simulink model "system_FIR_bank_decoder"  (Simulink 8.3)
settings: Solver=ode45  StartTime=0.0  StopTime=10  RelTol=1e-3
undefined symbols (not defined in the file or in its folder): fdesignblkfcn, gcbh
libraries: commutil2 x2
(part 2 of 2)

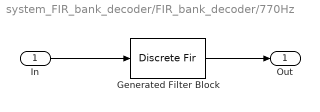
== system system_FIR_bank_decoder/FIR_bank_decoder/770Hz ==
  In : Inport
  Generated Filter Block : DiscreteFir  Tag=BlockMethodSubSystem  FilterStructure=Direct form symmetric  Coefficients=[0.021048100748084043 -0.02926286162127616 -0.014344339405233889 -0.0067382476342175519 -0.0033123904559366302 -0.0021945690276578204 -0.0021342071303361238 -0.0022934425052693599 -0.0021557510968869928 -0.001536841972853253 -0.0005235016935473541 0.00058759386859477594 0.0014491242644490197 0.0017708969698477183 0.0014585874915251354 0.00061878703844939242 -0.00044354826950585192 -0.00136089700455511 -0.0017988232627814934 -0.0016048306304633827 -0.00083332303586988873 0.0002421672794711616 0.0012517587307990547 0.001826200459492635 0.0017626470460959727 0.0010625791642325511 -2.6711098009971838e-05 -0.0011360179030814456 -0.0018571126120684983 -0.001935651064151669 -0.0013148457755932251 -0.00021185890996268823 0.0010052695934177559 0.0018872707487213719 0.0021248152733135744 0.0015951242710271173 0.00048699554077768256 -0.00084425051160600425 -0.0018964823074298872 -0.0023198333997277807 -0.0018939145551047107 -0.00080325835581027507 0.00064730516589957742 0.0018908439902302809 0.0024829039658738304 0.0022586425220235381 0.001118577978164267 -0.00038876585185248602 -0.0018239156066238533 -0.0026733845855196046 -0.0025850508415780015 -0.0015235746420565225 9.8462718731610923e-05 0.0017320698806078927 0.0028012826225293232 0.0029192523560542393 0.001972636913799473 0.0002734845029135913 -0.0015896954375363879 -0.0029233477215027909 -0.0032471603043519861 -0.0024101597386545605 -0.00068965280517628146 0.0013420758467165626 0.0029592478547132983 0.0035718941730886705 0.0029104506306473158 0.0011759708128102752 -0.0010476345159772472 -0.0029595495295805805 -0.0038642666267331735 -0.0033961128923412436 -0.0016942633995684863 0.00067242773425810838 0.0028625723334399292 0.0040920428977543402 0.003882971457832749 0.0022758252206261037 -0.00020302132854180453 -0.0026794330164426438 -0.0042706199501282589 -0.0043654735945765659 -0.0028983243153943477 -0.00033331843401783636 0.0024121533503752464 0.0043837819953542728 0.0048117339194579068 0.0035361082096169567 0.00094222332517836108 -0.0020601481562842537 -0.0043894290292150256 -0.005213252978909436 -0.0041781027657706582 -0.0016080612636526659 0.0015954691904100724 0.0043058302627674962 0.0055415888387755508 0.0048136835024899394 0.0023334413667720775 -0.0010362021330557435 -0.0041113741986643637 -0.0057862243907440408 -0.0054244151769606468 -0.0031030261300052128 0.00038481679566975817 0.0038081382852554664 0.0059389667376776919 0.0059894192755409513 0.0038935720589659611 0.00035523833276214235 -0.0033882281047023233 -0.005991540588728566 -0.0064993294746897032 -0.0046880882204626577 -0.0011646042858746047 0.0028465822396311108 0.0059164623818464962 0.0069265357518669985 0.0054720287743438879 0.0020301971526669846 -0.0022036194398257691 -0.0057212873206023158 -0.0072529382952613106 -0.0062136143169091882 -0.0029368435165044262 0.0014470907359265988 0.005384551681539747 0.0074587017277012273 0.0068995756468850332 0.0038548868599859731 -0.00061229573615546201 -0.0049387237433249449 -0.0075577428617720193 -0.007514679432755883 -0.0047852690650780341 -0.00030172072869157003 0.0043511265299573951 0.0075165351433368246 0.0080467150937750861 0.0057115794430851134 0.0013076313938961423 -0.0036156565354544738 -0.0073081930109354099 -0.0084400136036027733 -0.0065672305909212341 -0.0023245721628232432 0.0027968271489216224 0.0069794360967642098 0.00872015779915606 0.0073702080881285345 0.0033744958616032639 -0.0018647551369501331 -0.0064920262273558179 -0.0088511085597637752 -0.0080796097740328116 -0.0044191382710887022 0.00085345506904594228 0.0058715779690651079 0.0088409748695103384 0.0086860509306450791 0.0054356336329200059 0.00022143986170222401 -0.0051168645751970927 -0.0086748461106291707 -0.0091688916638644914 -0.0064015522032404909 -0.0013346529759097816 0.0042425490216516717 0.0083493712118810921 0.0095084847417085134 0.0072921448718452197 0.002465004547517967 -0.0032696589721588052 -0.00787137040913557 -0.0097013501466275687 -0.0080863506859156619 -0.0035909465012341248 ...(+5042 chars)]  InputProcessing=Columns as channels (frame based)
  Out : Outport
  wires:
  In/1 -> Generated Filter Block/1
  Generated Filter Block/1 -> Out/1

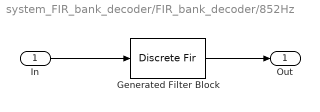
== system system_FIR_bank_decoder/FIR_bank_decoder/852Hz ==
  In : Inport
  Generated Filter Block : DiscreteFir  Tag=BlockMethodSubSystem  FilterStructure=Direct form symmetric  Coefficients=[0.023839593513569859 -0.026106670886814936 -0.014515913923892815 -0.0078635068286020057 -0.0045480316379694387 -0.0033125023745395172 -0.0030702773016210968 -0.0029641466005046573 -0.0024588534477011066 -0.0014330386067146878 -0.00011452378323294329 0.0010522474153322396 0.0016501906286755937 0.0014642374300596339 0.00060786967801007878 -0.00054209838800419775 -0.0014772482973398726 -0.0017921976058056773 -0.0013374155712994711 -0.00030506612887536638 0.00087472422424384356 0.0016866687577636987 0.0017817229796820561 0.0011008170041724777 -6.7951668830092398e-05 -0.0012338634266420179 -0.0018829581556778798 -0.0017310722292330893 -0.00081471251070362239 0.00047462403546293948 0.0015953679106102806 0.0020438242476589338 0.0016179295379949812 0.00046518805502698482 -0.00091654708573927243 -0.0019480212635727564 -0.0021464034237020165 -0.0014247206150643905 -3.7508109370541094e-05 0.0013906791174611499 0.0022706213384942465 0.0021899192012197204 0.0011001905319130917 -0.00042135809591145509 -0.0019045071189112523 -0.0025539731328647697 -0.002092463133230923 -0.00072009861981338775 0.0010000178906505223 0.0023770497455017541 0.0027529804807521294 0.0019202616543645158 0.00020435629835819638 -0.0016402729354980268 -0.0028262131054517343 -0.00281510525540949 -0.001583211314657491 0.00039262808518109873 0.0022694564801642417 0.0032224174937415602 0.0027848157683940233 0.0011074989164262419 -0.0011187022712652141 -0.0029195613294748721 -0.0034982347912125194 -0.0025584117004255574 -0.0004725215393152763 0.0018883392295170559 0.0034931229985446306 0.0036249270451743296 0.0021695195909299234 -0.00027888357370429843 -0.0026890375793498559 -0.0039958072741914418 -0.003597031588827398 -0.0016039092120171479 0.0011490864977044314 0.0034881849355724148 0.0043609149454591463 0.0033568320966274692 0.00083971336969076169 -0.0021067948801669501 -0.0042247171368122189 -0.0045502501148665933 -0.0028843693516404862 7.1967398731385661e-05 0.0030959780151318733 0.0048375524262719511 0.0045065369818951592 0.0022050002374939003 -0.0011215697125002667 -0.0040524937311592173 -0.0052801949618826649 -0.0042294902609412849 -0.0013093666776701719 0.0022536705603679683 0.0049270206978740223 0.0055144523843526656 0.0037058428394836007 0.0002355501063833989 -0.003415786161396827 -0.0056604358884984381 -0.0054892043449990078 -0.002920784864148521 0.00098471497505570656 0.0045496559355458384 0.0062074456351294436 0.0051917415254992003 0.0018893813508643899 -0.0023049838224737575 -0.0055797767405325197 -0.0064930396376156416 -0.0045954018879252453 -0.00065797037911517655 0.0036463250897162645 0.0064461224748369956 0.0064897427719319807 0.0037047375428177517 -0.00074460471538265606 -0.0049517196141328542 -0.0070744820626486475 -0.006158689233933555 -0.0025398425003342515 0.0022400377908260681 0.0061321131231064883 0.0074208299658351856 0.0054982560497843233 0.001156840977674564 -0.0037672796052483936 -0.0071289770683121961 -0.0074409759411050418 -0.0045249287379080828 0.00040422482224439075 0.0052351315586598411 0.0078578153585284211 0.0071062950474576865 0.0032608445674290544 -0.0020543345264128743 -0.0065522878586134672 -0.0082622360756481987 -0.0064084536760591389 -0.0017513523048681943 0.0037234866712307045 0.0076513455140711662 0.0083049672715876689 0.0053605338667787441 5.1003415149181457e-05 -0.0053414146508846995 -0.00847846955851159 -0.0079752044526672852 -0.0040080457338613424 0.0017406403995727327 0.0067924186865504525 0.0089517847692777534 0.0072490495502076386 0.0023900675486357285 -0.0035492195807516553 -0.0080034008198448317 -0.0090283068818453084 -0.0061482263646378699 -0.00057659715051141191 0.0052956996274064758 0.008921751675892188 0.0087164235545905654 0.0047329535394271607 -0.0013216208552966494 -0.0068503409744694278 -0.0094509499938668778 -0.0079763849798731006 -0.0030398229397014887 0.0032491107768218498 0.0081733712904150067 0.0095901393340554145 0.0068689647994716026 0.0011591458925277064 -0.005083069295184206 -0.0091558726262952802 ...(+5053 chars)]  InputProcessing=Columns as channels (frame based)
  Out : Outport
  wires:
  In/1 -> Generated Filter Block/1
  Generated Filter Block/1 -> Out/1

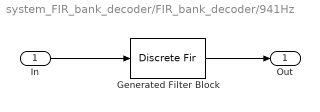
== system system_FIR_bank_decoder/FIR_bank_decoder/941Hz ==
  In : Inport
  Generated Filter Block : DiscreteFir  Tag=BlockMethodSubSystem  FilterStructure=Direct form symmetric  Coefficients=[0.025509633378811274 0.022027391281937769 -0.015629739982581058 0.01066284803954645 -0.0047831166861981292 0.0056878627848254123 -0.0019775559228465884 0.0012287487691349298 -0.0025670139817215295 -0.00089682443127405591 -0.0014324914095788913 0.00050888938642988039 0.0010653809095696922 0.0017962985083336011 0.0011208597776862796 0.00015952992258727708 -0.0010928572659544237 -0.0016584138927316103 -0.0014437839602567924 -0.00041506486813670373 0.00081415889396011182 0.0016601893507764819 0.0016336138422862543 0.00075543418376772622 -0.00054633853810124265 -0.0015869279553149694 -0.0018179488734876175 -0.0010935995063684118 0.0002287098190819126 0.0014648523119702398 0.0019647018619948432 0.001436416543403227 0.00013333133020686287 -0.0012817439544525135 -0.0020625248600068201 -0.0017768482585151014 -0.00053840721495798302 0.0010259408009693229 0.002099359380323892 0.0020903968392256421 0.00097089286371020275 -0.00071237104384959708 -0.0020702200555446438 -0.0023841595545743546 -0.0014492241416905142 0.00026574605147578482 0.0019094243426282453 0.0026117440970939744 0.0019437477009074892 0.00018307405317330571 -0.0017232791496264183 -0.0027566422826116386 -0.0023748863380560889 -0.0007350485104265801 0.0013836672211365495 0.0028332519276649142 0.0028108297305253749 0.0013174472467332816 -0.00092556264659052418 -0.0027826385279787064 -0.003201011718975369 -0.0019430086446150865 0.00037465411450848032 0.0025928002837349762 0.0035058400781362823 0.0025764007836806351 0.0002738990187042084 -0.0022695720481412168 -0.0036928074752020741 -0.0031870266537408873 -0.0009984174627757842 0.0018055402857457738 0.0037437476847058493 0.0037404939922762079 0.0017767189026404685 -0.0012058229600212691 -0.0036387020273276594 -0.0042045380891096995 -0.0025791591383506262 0.00048068760015451055 0.0033677770188416598 0.0045516701866640573 0.0033737188659410783 0.00035582322408828733 -0.0029178694320686886 -0.0047427881264862533 -0.0041115140023262496 -0.0012732346779163004 0.0023009278413217539 0.0047663412986232332 0.0047777260036137277 0.002253543599482365 -0.0015161883494841943 -0.0046015754267823717 -0.0053064217321209571 -0.0032372140061104667 0.00059142724660077957 0.0042051604868857196 0.0056766845822321475 0.0042018156960761926 0.00045171511976631551 -0.0036106993858542303 -0.005859781468159784 -0.0050775447330761317 -0.0015853396244687303 0.0028122744369163915 0.0058345648635002682 0.0058279044082092425 0.0027595622967925776 -0.0018328537806899094 -0.0055645182261874152 -0.0064236665849391394 -0.003925385001803978 0.00070013454311207706 0.0050431539301435254 0.0068180207947109743 0.0050311231388792035 0.00055595950578312282 -0.0042835843576532109 -0.0069750609934890288 -0.0060221129287031643 -0.001896624251093112 0.0033075635262751492 0.0068594085369391815 0.0068608579428576771 0.0032502975097536031 -0.0021319075260896121 -0.0064745520716545379 -0.0074940038004008887 -0.0045697271203565199 0.00078352658949030173 0.005820345492641303 0.0078682178156787227 0.0058072344641340295 0.00066912298961172348 -0.0049054770897861179 -0.0079698217689620626 -0.0068998037835217765 -0.002172008716647628 0.0037403534797150698 0.0077841828110188534 0.0077765126315403072 0.003698794600225258 -0.0023803062078963594 -0.0072885878984963208 -0.0084188750924269716 -0.005152502157324065 0.00086386672700348001 0.006489495104535406 0.0087789808308271645 0.0064792389847687223 0.00076217441800956534 -0.0054224346548773644 -0.0088146235301680403 -0.0076270280739622574 -0.0024244856601635164 0.0041053566776316349 0.0085308046712537829 0.0085368672595809367 0.0040564387482297324 -0.0025766252143383816 -0.0079289424423843423 -0.0091568569648412274 -0.0056065783056036631 0.00091675555196166388 0.0069992068855367785 0.0094768847001047499 0.0069880904510374077 0.00084457967604023609 -0.0058019139649227837 -0.0094385197591500703 -0.0081659172256053174 -0.0026052572843086688 0.0043467315054058295 0.0090666733847423724 0.0090679844972093356 0.0043234443682321471 ...(+5045 chars)]  InputProcessing=Columns as channels (frame based)
  Out : Outport
  wires:
  In/1 -> Generated Filter Block/1
  Generated Filter Block/1 -> Out/1
